simulink model "sample_serial_send"  (R2018a)
settings: Solver=ode4  StartTime=0.0  StopTime=10.0  FixedStep=0.001  RelTol=1e-3
undefined symbols (not defined in the file or in its folder): LF, serial
libraries: instrumentlib x2
settings Model: EnablePacing=on  Creator=shiib  LastModifiedBy=takada

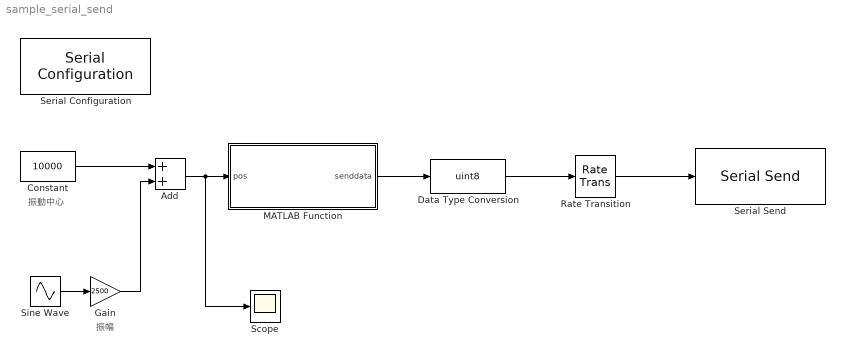
== system sample_serial_send ==
  note: 振幅
  note: 振動中心
  Add : Sum
  Constant : Constant  Value=10000  OutDataTypeStr=int16  SampleTime=1
  Data Type Conversion : DataTypeConversion  OutDataTypeStr=uint8
  Gain : Gain  Gain=2500  OutDataTypeStr=int16
  MATLAB Function : MATLAB Function  TreatAsAtomicUnit=on
  Rate Transition : RateTransition  OutPortSampleTime=0.075
  Scope : Scope
  Serial Configuration : instrumentlib/Serial Configuration  Priority=-200000  ComPortMenu=COM1  ComPort=COM1  ObjConstructor=serial('COM1');  BaudRate=115200  DataBits=8  Parity=none  StopBits=1  FlowControl=none  Timeout=10  ByteOrder=LittleEndian
  Serial Send : instrumentlib/Serial Send  ComPortMenu=COM1  ComPort=COM1  ObjConstructor=serial('COM1');  Terminator=LF ('\n')  EnableBlockingMode=on
  Sine Wave : Sin  Frequency=10  SampleTime=0
  wires:
  MATLAB Function/1(senddata) -> Data Type Conversion/1
  Sine Wave/1 -> Gain/1
  Constant/1 -> Add/1
  Gain/1 -> Add/2
  Add/1 -> Scope/1, MATLAB Function/1(pos)
  Data Type Conversion/1 -> Rate Transition/1
  Rate Transition/1 -> Serial Send/1

== matlab function sample_serial_send/MATLAB Function ==
  data: pos input; senddata output
% script_sendTargetPosition
% MATLAB EPOS LibraryのsendTargetPosition()から書き換え

% function [] = sendTargetPosition( obj, pos )

function senddata = func_sendTargetPosition(pos)
% pos = 20480;

%Sets the TargetPosition for Profile Position mode
%pos must be an integer.
pos_hex = '';

if pos >= 0
    pos_hex = dec2hex(pos, 8);
else
    pos_hex = dec2hex(2^32+pos, 8);
end

%% Build write object request frame EPOS Node 1
%opCode(write): 0x11
%Len-1: 3
%object index(Target Position): 0x607A
%subindex and nodeID: 0x0100
%BYTE Data[4]: pos_hex(1:4), pos_hex(5:8)


%opCode = uint16(myhex2dec('11'));
opCode = uint16(17);
Len_1 = uint16(3);
%DATA = uint16([myhex2dec('7A') myhex2dec('60') myhex2dec('00') myhex2dec('01') myhex2dec(pos_hex(7:8)) myhex2dec(pos_hex(5:6)) myhex2dec(pos_hex(3:4)) myhex2dec(pos_hex(1:2)) ]);
DATA = uint16([122 96 0 1 myhex2dec(pos_hex(7:8)) myhex2dec(pos_hex(5:6)) myhex2dec(pos_hex(3:4)) myhex2dec(pos_hex(1:2)) ]);
%DATAforCRC = uint16([myhex2dec('1103') myhex2dec('607A') myhex2dec('0100') myhex2dec(pos_hex(5:8)) myhex2dec(pos_hex(1:4)) myhex2dec('0000')]);
DATAforCRC = uint16([4355 24698 256 myhex2dec(pos_hex(5:8)) myhex2dec(pos_hex(1:4)) 0]);
numberofWordsCRC = 6;
crc_hex = dec2hex(CRCcalc(DATAforCRC, numberofWordsCRC),4);
CRC = uint16([myhex2dec(crc_hex(3:4)) myhex2dec(crc_hex(1:2))]);

% fwrite(obj, [opCode Len_1 DATA CRC char('O')]) %send all at once
% senddata=[opCode Len_1 DATA CRC char('O')];
senddata1=[opCode Len_1 DATA CRC 79];

% 16進数でsprintf
% sprintf('%x',senddata)

%% Controlword: Absolute Pos, start immediately EPOS Node 1
%Build write object request frame
%opCode(write): 0x11
%Len-1: 3
%object index(controlword): 0x6040
%subindex and nodeID: 0x0100
%device control command 0x003F

%opCode = uint16(myhex2dec('11'));
opCode = uint16(17);
Len_1 = uint16(3);
%DATA = uint16([myhex2dec('40') myhex2dec('60') myhex2dec('00') myhex2dec('01') myhex2dec('3F') myhex2dec('00') myhex2dec('00')  myhex2dec('00')]);
DATA = uint16([64,96,0,1,63,0,0,0]);
%DATAforCRC = uint16([myhex2dec('1103') myhex2dec('6040') myhex2dec('0100') myhex2dec('003F') myhex2dec('0000')  myhex2dec('0000')]);
%numberofWordsCRC = 6;
%crc_hex = dec2hex(CRCcalc(DATAforCRC, numberofWordsCRC),4);
%CRC = uint16([myhex2dec(crc_hex(3:4)) myhex2dec(crc_hex(1:2))]);
CRC = uint16([247,42]);

senddata2=[opCode Len_1 DATA CRC 79];

senddata=[senddata1 10 senddata2];
